simulink model "t2_sim_auto2"  (Simulink 7.3)
settings: Solver=ode45  StartTime=0.0  StopTime=8  RelTol=1e-3
values from neighbouring files (symbols this model uses):
  B = 5    [t1.m]
  K = 50    [t1.m]
  ka = 1053    [t1.m]
  ki = 5    [t1.m]
  ki2 = 1542    [t1.m]
  kp = 2547    [t1.m]
  kv = 0    [t1.m]
  M = 1    [t1.m]
  Ts = .02    (= 0.02)    [t1.m]
libraries: sdolib x1
settings Model: Creator=arash  LastModifiedBy=arash

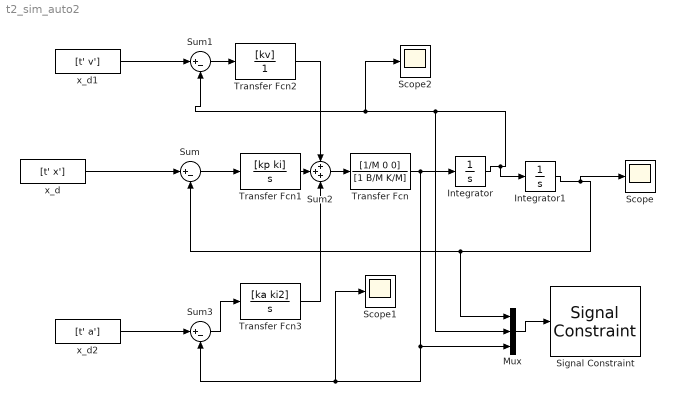
== system t2_sim_auto2 ==
  Integrator : Integrator
  Integrator1 : Integrator
  Mux : Mux  Inputs=3
  Scope : Scope
      settings: TimeRange=15
  Scope1 : Scope
      settings: TimeRange=15
  Scope2 : Scope
      settings: TimeRange=15  SaveName=ScopeData2
  Signal Constraint : sdolib/Signal Constraint  SystemSampleTime=-1  DialogPosition=[0.44296875 0.11375 0.45 0.31]  SaveIn=workspace  SaveAs=t2_sim_auto2_optim  LogID=SRO_DataLog_1
  Sum : Sum  Inputs=|+-  OutDataType=fixdt(1, 16)  OutScaling=2^0
  Sum1 : Sum  Inputs=|+-  OutDataType=fixdt(1, 16)  OutScaling=2^0
  Sum2 : Sum  Inputs=+++  OutDataType=fixdt(1, 16)  OutScaling=2^0
  Sum3 : Sum  Inputs=|+-  OutDataType=fixdt(1, 16)  OutScaling=2^0
  Transfer Fcn : TransferFcn  Numerator=[1/M 0 0]  Denominator=[1 B/M K/M]
  Transfer Fcn1 : TransferFcn  Numerator=[kp ki]  Denominator=[1 0]
  Transfer Fcn2 : TransferFcn  Numerator=[kv]  Denominator=1
  Transfer Fcn3 : TransferFcn  Numerator=[ka ki2]  Denominator=[1 0]
  x_d : FromWorkspace  VariableName=[t' x']  SampleTime=Ts
  x_d1 : FromWorkspace  VariableName=[t' v']  SampleTime=Ts
  x_d2 : FromWorkspace  VariableName=[t' a']  SampleTime=Ts
  wires:
  Sum/1 -> Transfer Fcn1/1
  x_d/1 -> Sum/1
  Transfer Fcn/1 -> Integrator/1, Sum3/2, Scope1/1, Mux/3
  Sum2/1 -> Transfer Fcn/1
  Transfer Fcn1/1 -> Sum2/2
  x_d1/1 -> Sum1/1
  Integrator1/1 -> Scope/1, Sum/2, Mux/1
  Integrator/1 -> Integrator1/1, Mux/2, Sum1/2, Scope2/1
  x_d2/1 -> Sum3/1
  Sum1/1 -> Transfer Fcn2/1
  Transfer Fcn3/1 -> Sum2/3
  Sum3/1 -> Transfer Fcn3/1
  Transfer Fcn2/1 -> Sum2/1
  Mux/1 -> Signal Constraint/1
